simulink model "model"  (R2022a)
settings: Solver=VariableStepAuto  StartTime=0.0  StopTime=20  RelTol=1e-3
undefined symbols (not defined in the file): B, I, lb, lc, lm, ln, Wb, Wc, Wn
settings Model: Creator=crist  LastModifiedBy=crist

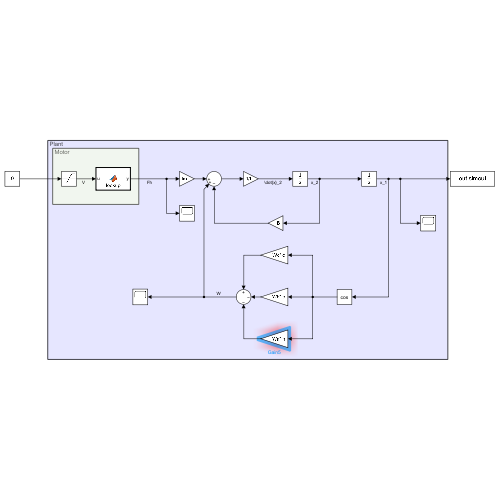
[thumbnail: Simulink's stored preview of the top-level diagram]
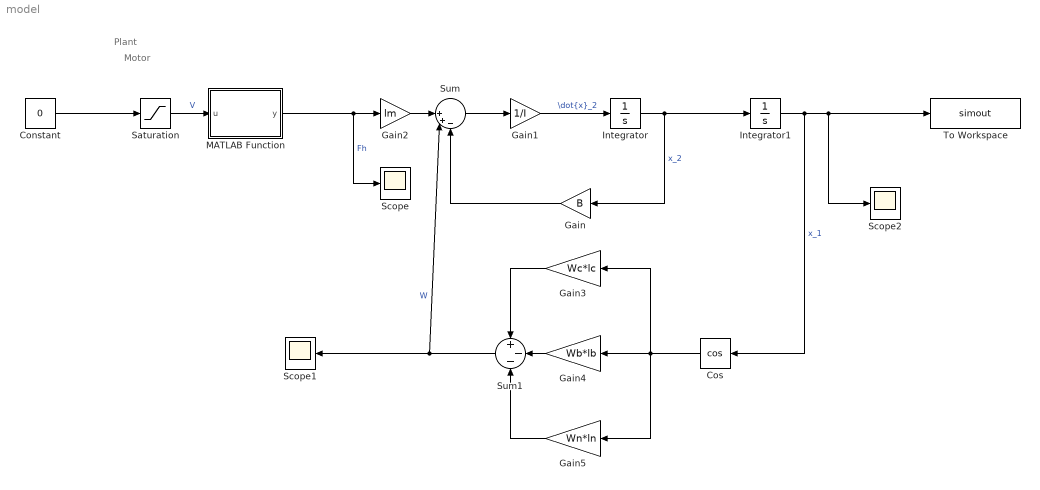
== system model ==
  note: Motor
  note: Plant
  Constant : Constant  Value=0
  Cos : Trigonometry  Operator=cos
  Gain : Gain  Gain=B
  Gain1 : Gain  Gain=1/I
  Gain2 : Gain  Gain=lm
  Gain3 : Gain  Gain=Wc*lc
  Gain4 : Gain  Gain=Wb*lb
  Gain5 : Gain  Gain=Wn*ln
  Integrator : Integrator
  Integrator1 : Integrator
  MATLAB Function : MATLAB Function  TreatAsAtomicUnit=on
  Saturation : Saturate  UpperLimit=6  LowerLimit=-6
  Scope : Scope
  Scope1 : Scope
  Scope2 : Scope
  Sum : Sum  Inputs=||++-
  Sum1 : Sum  Inputs=+--
  To Workspace : ToWorkspace  VariableName=simout  SaveFormat=Timeseries  SampleTime=-1
  wires:
  Cos/1 -> Gain5/1, Gain4/1, Gain3/1
  Gain5/1 -> Sum1/3
  Gain4/1 -> Sum1/2
  Sum1/1 -> Scope1/1, Sum/2  "W"
  Gain3/1 -> Sum1/1
  Integrator1/1 -> Scope2/1, To Workspace/1, Cos/1  "x_1"
  Sum/1 -> Gain1/1
  Gain2/1 -> Sum/1
  Integrator/1 -> Integrator1/1, Gain/1  "x_2"
  Gain1/1 -> Integrator/1  "\\dot{x}_2"
  Gain/1 -> Sum/3
  MATLAB Function/1(y) -> Scope/1, Gain2/1  "Fh"
  Constant/1 -> Saturation/1
  Saturation/1 -> MATLAB Function/1(u)  "V"

== matlab function model/MATLAB Function ==
  data: u input; y output
function y = lookup(u)
    dz = 2.369;

    if u < dz
        y = 0;
    else
        y = 0.0647*u-0.114;
    end
end
